simulink model "Animate_4link"  (R2014b)
settings: Solver=FixedStepDiscrete  StartTime=0.0  StopTime=tend  FixedStep=ts  RelTol=1e-3
InitFcn:
  | InitParams4
values from neighbouring files (symbols this model uses):
  tend = u(6)    [FallingRobotAnimate_3link.m]    (also in FallingRobotAnimate_4link.m = u(7); InitParams.m = q0_signal(end,1); InitParams4.m = q0_signal(end,1); SinusoidalPlanning.m = 1.2*num_cycles*T)
  tslow = 1.0/50.0    (= 0.02)    [InitParams.m]    (also in InitParams4.m)
settings Model: Creator=etreadwa  LastModifiedBy=Emma
settings DataIOCC: LimitDataPoints=off  SaveOutput=off  SignalLogging=off  DSMLogging=off  SaveTime=off
settings DebuggingCC: ArrayBoundsChecking=warning  ParameterUnderflowMsg=warning  UnnecessaryDatatypeConvMsg=warning  VectorMatrixConversionMsg=warning  SFcnCompatibilityMsg=warning
settings HardwareCC: ProdHWDeviceType=Generic->Unspecified (assume 32-bit Generic)

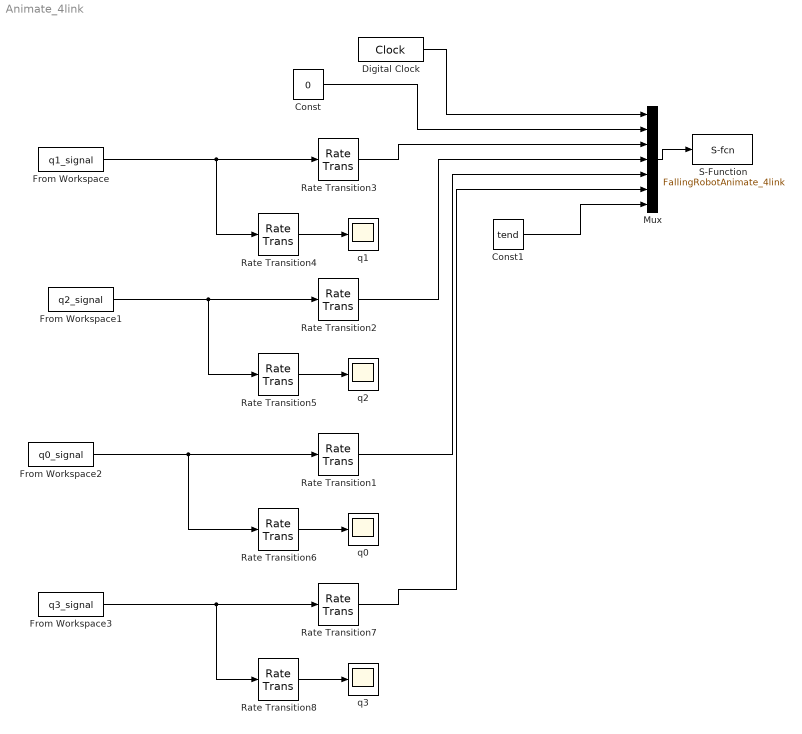
== system Animate_4link ==
  Const : Constant  Value=0
  Const1 : Constant  Value=tend
  Digital Clock : DigitalClock  SampleTime=tslow
  From Workspace : FromWorkspace  VariableName=q1_signal  SampleTime=0
  From Workspace1 : FromWorkspace  VariableName=q2_signal  SampleTime=0
  From Workspace2 : FromWorkspace  VariableName=q0_signal  SampleTime=0
  From Workspace3 : FromWorkspace  VariableName=q3_signal  SampleTime=0
  Mux : Mux  Inputs=7
  Rate Transition{1..8} (8 alike) : RateTransition
  S-Function : S-Function  FunctionName=FallingRobotAnimate_4link  Parameters=tslow  EnableBusSupport=off
  q{0..3} (4 alike) : Scope
      q0 settings: YMin=1.2  YMax=2.2  SaveName=q0  SampleInput=on  SampleTime=tsdata
      q1 settings: YMin=-700  YMax=900  SaveName=q1  SampleInput=on  SampleTime=tsdata
      q2 settings: YMin=-700  YMax=900  SaveName=q2  SampleInput=on  SampleTime=tsdata
      q3 settings: YMin=-700  YMax=900  SaveName=q3  SampleInput=on  SampleTime=tsdata
  wires:
  Mux/1 -> S-Function/1
  Digital Clock/1 -> Mux/1
  Const/1 -> Mux/2
  Rate Transition4/1 -> q1/1
  Rate Transition5/1 -> q2/1
  Rate Transition2/1 -> Mux/4
  Rate Transition6/1 -> q0/1
  From Workspace/1 -> Rate Transition4/1, Rate Transition3/1
  From Workspace1/1 -> Rate Transition5/1, Rate Transition2/1
  From Workspace2/1 -> Rate Transition6/1, Rate Transition1/1
  Rate Transition3/1 -> Mux/3
  Rate Transition1/1 -> Mux/5
  Rate Transition8/1 -> q3/1
  From Workspace3/1 -> Rate Transition8/1, Rate Transition7/1
  Rate Transition7/1 -> Mux/6
  Const1/1 -> Mux/7
